simulink model "matlab_follow_object_oldVersion"  (R2021b)
settings: Solver=FixedStepAuto  StartTime=0.0  StopTime=240  RelTol=1e-3  EnableMultiTasking=on
libraries: simulink x6, legoev3lib x6, simulink_extras x2
settings Model: ExtModeTrigDuration=2  Creator=s140  LastModifiedBy=s140
settings SolverCC: PositivePriorityOrder=on
settings OptimizationCC: EnhancedBackFolding=on  PassReuseOutputArgsAs=Individual arguments  ZeroExternalMemoryAtStartup=off  ZeroInternalMemoryAtStartup=off  MaxStackSize=64  OptimizeBlockOrder=speed  DifferentSizesBufferReuse=on  OptimizationCustomize=off  EfficientTunableParamExpr=on
settings DebuggingCC: ParameterTunabilityLossMsg=error
settings HardwareCC: ProdBitPerPointer=32  ProdBitPerSizeT=32  ProdBitPerPtrDiffT=32  ProdLargestAtomicInteger=Long  ProdWordSize=32  ProdHWDeviceType=ARM Compatible->ARM 9
settings SFSimCC: MATLABDynamicMemAlloc=off
settings RTWCC: Description=Embedded Coder  SystemTargetFile=ert.tlc  HardwareBoard=LEGO MINDSTORMS EV3  TLCOptions="-aInlineSetEventsForThisBaseRateFcn=TLC_FALSE -aSuppressMultiTaskScheduler=TLC_FALSE  -aRateBasedStepFcn=0"  TemplateMakefile=ert_default_tmf  Toolchain=Sourcery G++ Lite v2009q3
settings CodeAppCC: ForceParamTrailComments=on  IgnoreCustomStorageClasses=off  OperatorAnnotations=on  SimulinkDataObjDesc=on  SFDataObjDesc=on  InsertBlockDesc=on
settings ERTTargetCC: SupportContinuousTime=on  SupportVariableSizeSignals=on

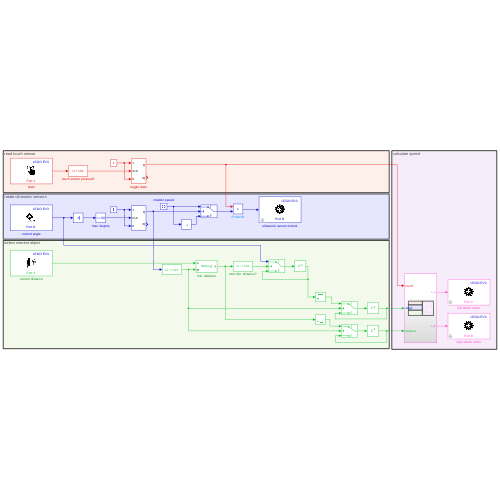
[thumbnail: Simulink's stored preview of the top-level diagram]
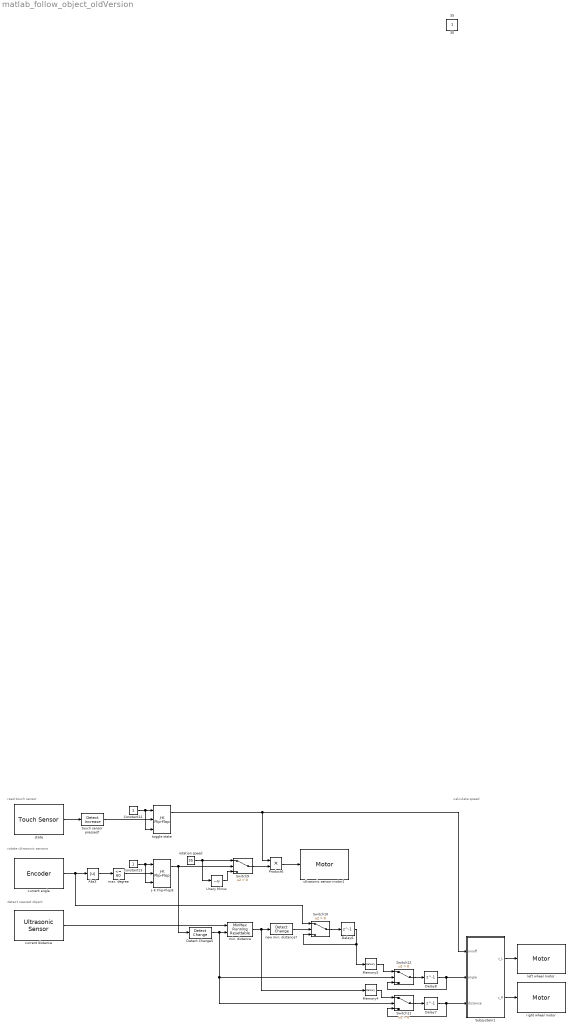
== system matlab_follow_object_oldVersion ==
  note: calculate speed
  note: detect nearest object
  note: rotate ultrasonic sensors
  note: read touch sensor
  Abs3 : Abs
  Constant12 : Constant  OutDataTypeStr=boolean
  Constant13 : Constant  OutDataTypeStr=boolean
  Delay6 : Delay  DelayLength=1
  Delay7 : Delay  DelayLength=1
  Delay8 : Delay  DelayLength=1
  Detect Change5 : simulink/Logic and Bit Operations/Detect Change  vinit=0  OutDataTypeStr=boolean
  J-K Flip-Flop9 : simulink_extras/Flip Flops/J-K Flip-Flop  initial_condition=0
  Memory4 : Memory
  Memory5 : Memory
  Product6 : Product
  Subsystem1 : Subsystem
  Switch{9..12} (4 alike) : Switch  Criteria=u2 > Threshold
  Unary Minus : UnaryMinus
  current angle : legoev3lib/Encoder  portNumber=D  opMode=No reset  sampleTime=0.005
      settings: SourceProductBaseCode=LEGOEV3
  current distance : legoev3lib/Ultrasonic Sensor  PortNumber=4  sampleTime=0.005
      settings: SourceProductBaseCode=LEGOEV3
  left wheel motor : legoev3lib/Motor  sportNumber=A  sstopAction=Brake
  max. degree : simulink/Logic and Bit Operations/Compare To Constant  relop=<=  const=60  OutDataTypeStr=boolean
  min. distance : simulink/Math Operations/MinMax Running Resettable  Function=min  vinit=160.0
  new min. distance? : simulink/Logic and Bit Operations/Detect Change  vinit=0  OutDataTypeStr=boolean
  right wheel motor : legoev3lib/Motor  sportNumber=B  sstopAction=Brake
  rotation speed : Constant  Value=35
  state : legoev3lib/Touch Sensor  portNumber=1  sampleTime=0.005
      settings: SourceProductBaseCode=LEGOEV3
  toggle state : simulink_extras/Flip Flops/J-K Flip-Flop  initial_condition=0
  touch sensor pressed? : simulink/Logic and Bit Operations/Detect Increase  vinit=0.0  OutDataTypeStr=boolean
  ultrasonic sensor motor1 : legoev3lib/Motor  sportNumber=D  sstopAction=Brake
  30 : Constant  IOType=siggen
  35 : Constant  IOType=siggen
  wires:
  toggle state/1 -> Subsystem1/1(on/off), Product6/1
  Subsystem1/2(v_R) -> right wheel motor/1
  Constant13/1 -> J-K Flip-Flop9/3, J-K Flip-Flop9/1
  Switch11/1 -> Delay7/1
  touch sensor pressed?/1 -> toggle state/2
  state/1 -> touch sensor pressed?/1
  Subsystem1/1(v_L) -> left wheel motor/1
  new min. distance?/1 -> Switch10/2
  Delay6/1 -> Memory5/1, Switch10/3
  Delay7/1 -> Switch11/3, Subsystem1/3(distance)
  Memory4/1 -> Switch11/1
  Delay8/1 -> Switch12/3, Subsystem1/2(angle)
  rotation speed/1 -> Switch9/1, Unary Minus/1
  max. degree/1 -> J-K Flip-Flop9/2
  Abs3/1 -> max. degree/1
  Switch9/1 -> Product6/2
  Constant12/1 -> toggle state/3, toggle state/1
  current angle/1 -> Abs3/1, Switch10/1
  Detect Change5/1 -> min. distance/2, Switch12/2, Switch11/2
  min. distance/1 -> new min. distance?/1, Memory4/1
  Memory5/1 -> Switch12/1
  Product6/1 -> ultrasonic sensor motor1/1
  Switch10/1 -> Delay6/1
  current distance/1 -> min. distance/1
  Switch12/1 -> Delay8/1
  J-K Flip-Flop9/1 -> Switch9/2, Detect Change5/1
  Unary Minus/1 -> Switch9/3

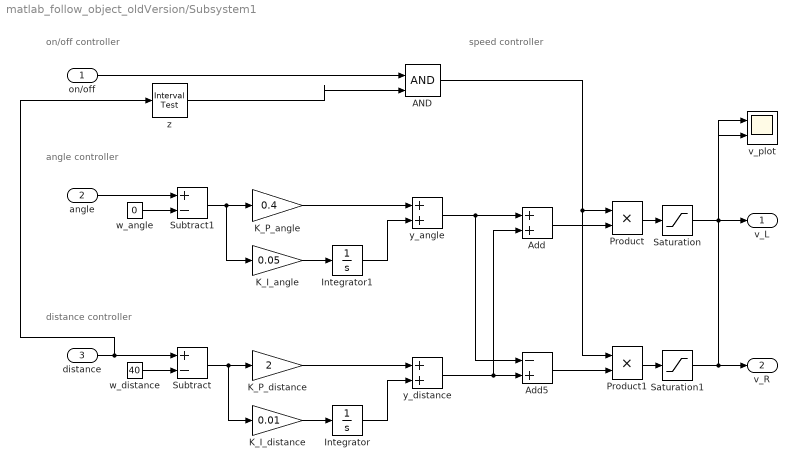
== system matlab_follow_object_oldVersion/Subsystem1 ==
  note: speed controller
  note: distance controller
  note: angle controller
  note: on/off controller
  on/off : Inport  Description=On/Off
  angle : Inport  Port=2
  distance : Inport  Port=3
  AND : Logic  IconShape=distinctive  AllPortsSameDT=off  OutDataTypeStr=boolean
  Add : Sum
  Add5 : Sum  Inputs=-+
  Integrator : Integrator  LimitOutput=on  UpperSaturationLimit=200  LowerSaturationLimit=-200
  Integrator1 : Integrator  LimitOutput=on  UpperSaturationLimit=200  LowerSaturationLimit=-200
  K_I_angle : Gain  Gain=0.05
  K_I_distance : Gain  Gain=0.01
  K_P_angle : Gain  Gain=0.4
  K_P_distance : Gain  Gain=2
  Product : Product
  Product1 : Product
  Saturation : Saturate  UpperLimit=100  LowerLimit=-100
  Saturation1 : Saturate  UpperLimit=100  LowerLimit=-100
  Subtract : Sum  Inputs=+-
  Subtract1 : Sum  Inputs=+-
  v_plot : Scope  NumInputPorts=2
  w_angle : Constant  Value=0
  w_distance : Constant  Value=40
  y_angle : Sum
  y_distance : Sum
  z : simulink/Logic and Bit Operations/Interval Test  IntervalClosedRight=on  uplimit=150  IntervalClosedLeft=on  lowlimit=25  OutDataTypeStr=boolean
  v_L : Outport
  v_R : Outport  Port=2
  wires:
  y_distance/1 -> Add/2, Add5/2
  Add5/1 -> Product1/2
  Product1/1 -> Saturation1/1
  Integrator1/1 -> y_angle/2
  Product/1 -> Saturation/1
  K_P_distance/1 -> y_distance/1
  Saturation1/1 -> v_R/1, v_plot/2
  K_P_angle/1 -> y_angle/1
  K_I_angle/1 -> Integrator1/1
  y_angle/1 -> Add/1, Add5/1
  Subtract1/1 -> K_P_angle/1, K_I_angle/1
  Saturation/1 -> v_L/1, v_plot/1
  distance/1 -> z/1, Subtract/1
  angle/1 -> Subtract1/1
  K_I_distance/1 -> Integrator/1
  Add/1 -> Product/2
  Subtract/1 -> K_P_distance/1, K_I_distance/1
  Integrator/1 -> y_distance/2
  w_distance/1 -> Subtract/2
  w_angle/1 -> Subtract1/2
  AND/1 -> Product1/1, Product/1
  on/off/1 -> AND/1
  z/1 -> AND/2
